simulink model "dataIdent"  (Simulink 7.2)
settings: Solver=ode1  StartTime=0.0  StopTime=100  FixedStep=0.002  RelTol=1e-3
libraries: simulink x1
settings Model: Creator=Aluno  LastModifiedBy=Aluno  ExtModeTrigDuration=5000
settings SolverCC: PositivePriorityOrder=on
settings RTWCC: SystemTargetFile=quarc_windows.tlc  TemplateMakefile=quarc_default_tmf  Description=QUARC Win32 Target  ProcessScript=quarc_windows_make_rtw_hook
settings STFCustomTargetCC: TargetPreCompLibLocation=C:\DOCUME~1\ALLUSE~1\DADOSD~1\QUARC\lib\2008b\windows\release  SystemTargetFile=quarc_windows.tlc
settings GRTTargetCC: TargetPreCompLibLocation=C:\DOCUME~1\ALLUSE~1\DADOSD~1\QUARC\lib\2008b\windows\release  CompOptLevelCompliant=off  MatFileLogging=off  ExtMode=on  ExtModeMexFile=quarc_comm

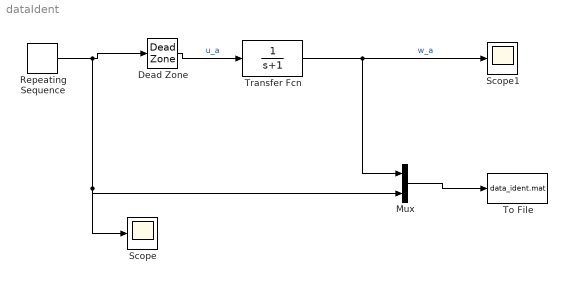
== system dataIdent ==
  Dead Zone : DeadZone  SaturateOnIntegerOverflow=on
  Mux : Mux  Inputs=2
  Repeating Sequence : simulink/Sources/Repeating Sequence  SystemSampleTime=-1  rep_seq_t=[0 1 2 3 4]*10  rep_seq_y=[0 1 0 -1 0]
  Scope : Scope
      settings: YMin=-1  YMax=0.3
  Scope1 : Scope
      settings: YMin=-0.45  YMax=0
  To File : ToFile  Filename=data_ident.mat
  Transfer Fcn : TransferFcn  Denominator=[1 1]
  wires:
  Dead Zone/1 -> Transfer Fcn/1  "u_a"
  Transfer Fcn/1 -> Scope1/1, Mux/1  "w_a"
  Mux/1 -> To File/1
  Repeating Sequence/1 -> Dead Zone/1, Scope/1, Mux/2
